simulink library "VariousBlocksLibrary"  (R2015b)
settings: Solver=ode45  StartTime=0.0  StopTime=10.0  RelTol=1e-3
undefined symbols (not defined in the file or in its folder): LopesParams
undefined symbols (not defined in the file): LopesParamsSendDataArrayLen
libraries: simulink x17, dspmtrx3 x9, LopesDevelopmentLibrary x2, LopesLibrary x1, VariousBlocksLibrary x1
(part 2 of 2)

== system VariousBlocksLibrary/Various/Stopwatch ==
  note: Stopwatch -
      | Outputs time in seconds.
      | Reset during high level of Rest pulse
  ResetHighActive : Inport
  Counter Free-Running : simulink/Sources/Counter Free-Running  NumBits=32  tsamp=-1
  Data Type Conversion : DataTypeConversion  OutDataTypeStr=double
  Gain : Gain  Gain=LopesParams.ts
  Latch : VariousBlocksLibrary/Various/Latch  ic=0
  Subtract : Sum  Inputs=+-
  Time_s : Outport
  wires:
  ResetHighActive/1 -> Latch/Enable
  Data Type Conversion/1 -> Gain/1
  Gain/1 -> Time_s/1
  Latch/1 -> Subtract/2  "startTime"
  Subtract/1 -> Data Type Conversion/1
  Counter Free-Running/1 -> Subtract/1, Latch/1

== system VariousBlocksLibrary/Various/TriggerAtPhaseCrossing ==
  Phase : Inport
  PhaseToTrigger : Inport  Port=2
  Detect Rise Nonnegative : simulink/Logic and Bit Operations/Detect Rise Nonnegative  vinit=0  InputProcessing=Inherited  OutDataTypeStr=boolean
  PhaseWrapperAroundZero : LopesDevelopmentLibrary/Various/PhaseWrapperAroundZero
  Subtract : Sum  Inputs=+-
  Trigger : Outport
  wires:
  Detect Rise Nonnegative/1 -> Trigger/1
  Phase/1 -> Subtract/1
  Subtract/1 -> PhaseWrapperAroundZero/1
  PhaseToTrigger/1 -> Subtract/2
  PhaseWrapperAroundZero/1 -> Detect Rise Nonnegative/1

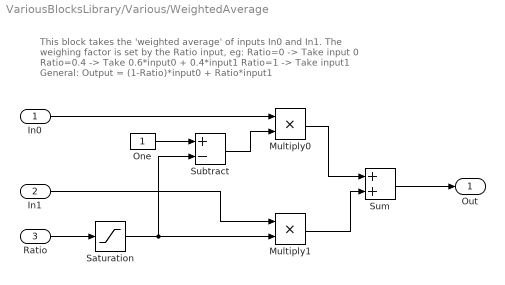
== system VariousBlocksLibrary/Various/WeightedAverage ==
  note: This block takes the 'weighted average' of inputs In0 and In1.
      | The weighing factor is set by the Ratio input, eg:
      | Ratio=0 -> Take input 0
      | Ratio=0.4 -> Take 0.6*input0  + 0.4*input1
      | Ratio=1 -> Take input1
      | General: Output = (1-Ratio)*input0 + Ratio*input1
  In0 : Inport
  In1 : Inport  Port=2
  Ratio : Inport  Port=3
  Multiply0 : Product  Inputs=**
  Multiply1 : Product  Inputs=**
  One : Constant
  Saturation : Saturate  UpperLimit=1  LowerLimit=0
  Subtract : Sum  Inputs=+-
  Sum : Sum
  Out : Outport
  wires:
  Ratio/1 -> Saturation/1
  In1/1 -> Multiply1/1
  Multiply1/1 -> Sum/2
  Subtract/1 -> Multiply0/2
  Saturation/1 -> Multiply1/2, Subtract/2
  Sum/1 -> Out/1
  Multiply0/1 -> Sum/1
  One/1 -> Subtract/1
  In0/1 -> Multiply0/1

== system VariousBlocksLibrary/Various/GenerateSyncPulseFromPhase/DetectPhaseSignalReset ==
  note: This block detects the event of phase reset (i.e., when it
      | goes from (approximately) 100 to (approximately) 0.
      | It does this by checking whether there is a decrease of at
      | least 50% within one sample time.
  Phase : Inport
  Compare To Constant : simulink/Logic and Bit Operations/Compare To Constant  relop=<  const=-50  OutDataTypeStr=boolean
  Subtract : Sum  Inputs=+-
  Unit Delay : UnitDelay  SampleTime=-1
  PhaseReset : Outport
  wires:
  Phase/1 -> Subtract/1, Unit Delay/1
  Compare To Constant/1 -> PhaseReset/1
  Unit Delay/1 -> Subtract/2
  Subtract/1 -> Compare To Constant/1

== system VariousBlocksLibrary/Various/GenerateSyncPulseFromPhase/GenerateRandomValue ==
  note: Generate a uniform random number between Minimum and Maximum each
      | time Trigger rises.
  Maximum : Inport
  Minimum : Inport  Port=2
  Trigger : TriggerPort  PortDimensions=1
  Add : Sum
  Product : Product  RndMeth=Zero
  Subtract : Sum  Inputs=+-
  Uniform Random Number : UniformRandomNumber  Minimum=0  Seed=66
  Out : Outport  InitialOutput=0
  wires:
  Maximum/1 -> Subtract/1
  Uniform Random Number/1 -> Product/1
  Product/1 -> Add/1
  Subtract/1 -> Product/2
  Add/1 -> Out/1
  Minimum/1 -> Add/2, Subtract/2

== matlab function VariousBlocksLibrary/StringFunctions/strlen ==
  data: s input; len output
function len = strlen(s)
%#codegen

% This function returns the length of the actual string, WITHOUT any
% trailing '\0's. So, the array  ['h','e','l','l','o',0,0,0,0] returns 5.
%
% s should be a uint8-array containing a string terminated with at least
% one '\0' character. The ASCII Encode block generates such an array
% (the array generated is fixed length, the first n bytes are the string,
% all other bytes are '\0'). 
%
% If the string does not have a trailing '\0' (in other words, if it is
% too large for its containing array), it returns the length of the array.

len = uint32(1);
maxlen = length(s);

while (len<= maxlen && s(len)~=0), 
    len = len + 1; 
end;
% Now len is the index of the first trailing '\0' (or maxlen+1);
% that is one more than the string length, so decrease by one:
len = len - 1;

== matlab function VariousBlocksLibrary/StringFunctions/concat ==
  data: s1 input; s1_len input; y output; s2 input; s2_len input; y_len output
function [y,y_len]= concat(s1,s1_len, s2, s2_len)
%#codegen

% Concatenates s1 and s2 into y, using a specified delimiter.
%
% s1 and s2 should be uint8-arrays containing a (possibly null-terminated) string.
% Usually, they will be a fixed-length array, holding the string in the
% first part; padded with zeros.
% s1_len and s2_len should be the actual string length (thus, the array
% uint8(['h','o','i',0,0,0,0]) has length 3. Use the strlen block for
% this.
%
% The result of this function is a fixed-length uint8-array, holding the
% string in the first part, padded with zeros, and the length of the
% resulting string (trailing zeros are not counted)
%
% If the resulting string would be too large to fit in the output array,
% it is truncated such that the output array is null-terminated and has
% maximum length.
%
% If s1_len> length(s1) (or similar with s2), the full length of the array
% will be taken as string.

%% Parameters
outputArrayLength = uint32(100); % The maximum string length is one less because of the trailing null-char
delimiter = uint8('; '); % Examples: uint8(';'), uint8('; ')
                        % Cannot be a non-empty string (if you don't want a delimiter, remove it from the Add() lines.


%% The work itself

i = uint32(1); % index within y
delimiter_len = length(delimiter);
y=zeros(outputArrayLength,1);

[y,i] = Add(s1, s1_len,              y, i, outputArrayLength);
[y,i] = Add(delimiter,delimiter_len, y, i, outputArrayLength);
[y,i] = Add(s2, s2_len,              y, i, outputArrayLength);

y_len = i-1;

%-------------------------------------------------
%% This subfunction actually adds the given string. If the output string
% is alrady 'full', nothing happens.
function [y, i] = Add(whichArray, stringLength, y, i, outputArrayLength)
nToCopy = min([length(whichArray),stringLength, outputArrayLength - i]);
if (nToCopy~=0),
    y(i:(i+nToCopy-1)) = whichArray(1:nToCopy);
    i = i + nToCopy;
end;

== matlab function VariousBlocksLibrary/StringFunctions/concat3 ==
  data: s1 input; s1_len input; y output; s2 input; s2_len input; y_len output; s3 input; s3_len input
function [y,y_len]= concat3(s1,s1_len, s2, s2_len,s3,s3_len)
%#codegen

% Concatenates s1 and s2, ... into y, using a specified delimiter.
%
% s1 and s2 should be uint8-arrays containing a (possibly null-terminated) string.
% Usually, they will be a fixed-length array, holding the string in the
% first part; padded with zeros.
% s1_len and s2_len should be the actual string length (thus, the array
% uint8(['h','o','i',0,0,0,0]) has length 3. Use the strlen block for
% this.
%
% The result of this function is a fixed-length uint8-array, holding the
% string in the first part, padded with zeros, and the length of the
% resulting string (trailing zeros are not counted)
%
% If the resulting string would be too large to fit in the output array,
% it is truncated such that the output array is null-terminated and has
% maximum length.
%
% If s1_len> length(s1) (or similar with s2), the full length of the array
% will be taken as string.

%% Parameters
outputArrayLength = uint32(100); % The maximum string length is one less because of the trailing null-char
delimiter = uint8(';'); % Examples: uint8(';'), uint8('; ')
                        % Cannot be a non-empty string (if you don't want a delimiter, remove it from the Add() lines.


%% The work itself

i = uint32(1); % index within y
delimiter_len = length(delimiter);
y=zeros(outputArrayLength,1);

[y,i] = Add(s1, s1_len,              y, i, outputArrayLength);
[y,i] = Add(delimiter,delimiter_len, y, i, outputArrayLength);
[y,i] = Add(s2, s2_len,              y, i, outputArrayLength);
[y,i] = Add(delimiter,delimiter_len, y, i, outputArrayLength);
[y,i] = Add(s3, s3_len,              y, i, outputArrayLength);

y_len = i-1;

%-------------------------------------------------
%% This subfunction actually adds the given string. If the output string
% is alrady 'full', nothing happens.
function [y, i] = Add(whichArray, stringLength, y, i, outputArrayLength)
nToCopy = min([length(whichArray),stringLength, outputArrayLength - i]);
if (nToCopy~=0),
    y(i:(i+nToCopy-1)) = whichArray(1:nToCopy);
    i = i + nToCopy;
end;

== matlab function VariousBlocksLibrary/StringFunctions/Pad/pad ==
  data: s input uint8; outArrayLen parameter; y output uint8; y_len output
function [y,y_len]= pad(s,outArrayLen)
%#codegen

% Given s, being an any-(fixed!)-length uint8-array, it outputs
% a 'string' array consisting of a default size (outArrayLen, as a
% parameter),padded with zero's
% together with a length indicating the number of 'valid' bytes in the
% string.
%
% If the string s is too long, it will use the first outputLen-1 chars (and
% add a null-char to fill the whole string up).

y = uint8(zeros(1,outArrayLen));
y_len = min(length(s), outArrayLen-1);
for i=1:y_len,
    y(i) = s(i);
end;

== matlab function VariousBlocksLibrary/StringFunctions/concatWithOptionalDelimiter ==
  data: s1 input; s1_len input; y output uint8; s2 input; s2_len input; y_len output; outputArrayLength parameter
function [y,y_len]= concatWithOptionalDelimiter(s1,s1_len, s2, s2_len, outputArrayLength)
%#codegen

% Concatenates s1 and s2 into y, using a specified delimiter if both strings are non-empty.
%
% s1 and s2 should be uint8-arrays containing a (possibly null-terminated) string.
% Usually, they will be a fixed-length array, holding the string in the
% first part; padded with zeros.
% s1_len and s2_len should be the actual string length (thus, the array
% uint8(['h','o','i',0,0,0,0]) has length 3. Use the strlen block for
% this.
%
% The result of this function is a fixed-length uint8-array, holding the
% string in the first part, padded with zeros, and the length of the
% resulting string (trailing zeros are not counted)
%
% If the resulting string would be too large to fit in the output array,
% it is truncated such that the output array is null-terminated and has
% maximum length.
%
% If s1_len> length(s1) (or similar with s2), the full length of the array
% will be taken as string.
%
% Note on outputArrayLength: The maximum string length is one less because of the trailing null-char

%% Parameters
delimiter = uint8(';'); % Examples: uint8(';'), uint8('; ')
                        % Cannot be a non-empty string (if you don't want a delimiter, remove it from the Add() lines.


%% The work itself

i = 1; % index within y
delimiter_len = length(delimiter);
y=uint8(zeros(outputArrayLength,1));

[y,i] = Add(s1, s1_len,              y, i, outputArrayLength);
if (s1_len~=0 && s2_len ~=0)
    [y,i] = Add(delimiter,delimiter_len, y, i, outputArrayLength);
end;
[y,i] = Add(s2, s2_len,              y, i, outputArrayLength);

y_len = i-1;

%-------------------------------------------------
%% This subfunction actually adds the given string. If the output string
% is alrady 'full', nothing happens.
function [y, i] = Add(whichArray, stringLength, y, i, outputArrayLength)
nToCopy = min([length(whichArray),stringLength, outputArrayLength - i]);
if (nToCopy~=0),
    y(i:(i+nToCopy-1)) = whichArray(1:nToCopy);
    i = i + nToCopy;
end;

== matlab function VariousBlocksLibrary/StringFunctions/ShowStringInMatlabConsoleIfNotEmpty ==
  data pre settings: description=Small string that is put in front of the received text.
  data: stringArray input; len input; pre input; enable input
function fcn(stringArray,len, pre, enable)
%#codegen
persistent t;
if isempty(t)
    t = 0;
end;
t = t+1;
    
coder.extrinsic('fprintf');
if (len~=0 && enable)
    fprintf('%6d: %s  (len = %d) - *%s*\n', t,char(pre'),len,char(stringArray(1:len).')); 
%    feval ('AddToGlobalXX',len);
end;

== matlab function VariousBlocksLibrary/StringFunctions/concatDelimiter ==
  data: s1 input; s1_len input; y output; s2 input; s2_len input; y_len output
function [y,y_len]= concatDelimiter(s1,s1_len, s2, s2_len)
%#codegen

% Concatenates s1 and s2 into y, using a ';' as a delimiter.
%
% s1 and s2 should be uint8-arrays containing a (possibly null-terminated) string.
% Usually, they will be a fixed-length array, holding the string in the
% first part; padded with zeros.
% s1_len and s2_len should be the actual string length (thus, the array
% uint8(['h','o','i',0,0,0,0]) has length 3. Use the strlen block for
% this.
%
% The result of this function is a fixed-length uint8-array, holding the
% string in the first part, padded with zeros, and the length of the
% resulting string (trailing zeros are not counted)
%
% If the resulting string would be too large to fit in the output array,
% it is truncated such that the output array is null-terminated and has
% maximum length.
%
% If s1_len> length(s1) (or similar with s2), the full length of the array
% will be taken as string.

%% Parameters
outputArrayLength = uint32(100); % The maximum string length is one less because of the trailing null-char
delimiter = uint8(';'); % Examples: uint8(';'), uint8('; ')
                        % Cannot be a non-empty string (if you don't want a delimiter, remove it from the Add() lines.
delimiter_len = 1;


%% The work itself
i = uint32(1); % index within y
y=zeros(outputArrayLength,1);

[y,i] = Add(s1, s1_len,              y, i, outputArrayLength);
[y,i] = Add(delimiter,delimiter_len, y, i, outputArrayLength);
[y,i] = Add(s2, s2_len,              y, i, outputArrayLength);

y_len = i-1;

%-------------------------------------------------
%% This subfunction actually adds the given string. If the output string
% is alrady 'full', nothing happens.
function [y, i] = Add(whichArray, stringLength, y, i, outputArrayLength)
nToCopy = min([length(whichArray),stringLength, outputArrayLength - i]);
if (nToCopy~=0),
    y(i:(i+nToCopy-1)) = whichArray(1:nToCopy);
    i = i + nToCopy;
end;

== matlab function VariousBlocksLibrary/StringFunctions/strlen_as_double ==
  data: s input; len output
function len = strlen(s)
%#codegen

% This function returns the length of the actual string, WITHOUT any
% trailing '\0's. So, the array  ['h','e','l','l','o',0,0,0,0] returns 5.0.
% The output of this function is a double.
%
% s should be a uint8-array containing a string terminated with at least
% one '\0' character. The ASCII Encode block generates such an array
% (the array generated is fixed length, the first n bytes are the string,
% all other bytes are '\0'). 
%
% If the string does not have a trailing '\0' (in other words, if it is
% too large for its containing array), it returns the length of the array.

len = 1.0;
maxlen = length(s);

while (len<= maxlen && s(len)~=0), 
    len = len + 1; 
end;
% Now len is the index of the first trailing '\0' (or maxlen+1);
% that is one more than the string length, so decrease by one:
len = len - 1;

== matlab function VariousBlocksLibrary/StringFunctions/concat5/concat5 ==
  data: s1 input; s1_len input; y output size=outStrLen; s2 input; s2_len input; y_len output; s3 input; s3_len input; s4 input; s4_len input; s5 input; s5_len input size=1; outStrLen parameter
function [y,y_len]= concat5(s1,s1_len, s2, s2_len,s3,s3_len, s4, s4_len, s5, s5_len, outStrLen)
%#codegen

% Concatenates s1 and s2, ... into y, using a specified delimiter.
%
% s1 and s2 should be uint8-arrays containing a (possibly null-terminated) string.
% Usually, they will be a fixed-length array, holding the string in the
% first part; padded with zeros.
% s1_len and s2_len should be the actual string length (thus, the array
% uint8(['h','o','i',0,0,0,0]) has length 3. Use the strlen block for
% this.
%
% The result of this function is a fixed-length uint8-array, holding the
% string in the first part, padded with zeros, and the length of the
% resulting string (trailing zeros are not counted)
%
% If the resulting string would be too large to fit in the output array,
% it is truncated such that the output array is null-terminated and has
% maximum length.
%
% If s1_len> length(s1) (or similar with s2), the full length of the array
% will be taken as string.

%% Parameters
outputArrayLength = uint32(outStrLen); % The maximum string length is one less because of the trailing null-char


%% The work itself

i =uint32(1); % index within y
y=uint8(zeros(outputArrayLength,1));

[y,i] = Add(s1, s1_len, y, i, outputArrayLength);
[y,i] = Add(s2, s2_len, y, i, outputArrayLength);
[y,i] = Add(s3, s3_len, y, i, outputArrayLength);
[y,i] = Add(s4, s4_len, y, i, outputArrayLength);
[y,i] = Add(s5, s5_len, y, i, outputArrayLength);

y_len = double(i-1);

%-------------------------------------------------
%% This subfunction actually adds the given string. If the output string
% is alrady 'full', nothing happens.
function [y, i] = Add(whichArray, stringLength, y, i, outputArrayLength)
nToCopy = min([length(whichArray),stringLength, outputArrayLength - i]);
if (nToCopy~=0),
    y(i:(i+nToCopy-1)) = whichArray(1:nToCopy);
    i = i + nToCopy;
end;

== matlab function VariousBlocksLibrary/Various/RateLimiterWithReset/RateLimiterWithReset ==
  data: u input; y output; rate input; initialValue input; reset_high_active input; ts parameter; y_is_u output double
function [y,y_is_u] = RateLimiterWithReset(u, rate, initialValue, reset_high_active, ts)
%#codegen

% Note: rate should be positive!

persistent currentValue;

if isempty(currentValue)
    currentValue = initialValue;
end;

% For safety, prevent negative rate (if the rate is negative, signals grow
% out of bounds; it is better to set the rate to 0 in those cases, which
% will keep the signals fixed. Not what we want, but not dangerous either).
if rate<0,
    rate = 0;
end;

if reset_high_active,
    currentValue = initialValue;
else
    % Rate-limit
    if currentValue < u,
        currentValue = min(currentValue + rate*ts, u);
    elseif currentValue > u,
        currentValue = max(currentValue - rate*ts, u);
    %else
        % currentValue is alreay equal to u, so don't do anything
    end;
end;
y = currentValue;

if y == u,
    y_is_u = 1;
else
    y_is_u = 0;
end;

== matlab function VariousBlocksLibrary/StringFunctions/PadStrAsDouble/pad ==
  data: s input uint8; outArrayLen parameter; y output uint8; y_len output
function [y,y_len]= pad(s,outArrayLen)
%#codegen

% Given s, being an any-(fixed!)-length uint8-array, it outputs
% a 'string' array consisting of a default size (outArrayLen, as a
% parameter),padded with zero's
% together with a length indicating the number of 'valid' bytes in the
% string.
%
% If the string s is too long, it will use the first outputLen-1 chars (and
% add a null-char to fill the whole string up).

y = uint8(zeros(1,outArrayLen));
y_len = min(length(s), outArrayLen-1);
for i=1:y_len,
    y(i) = s(i);
end;
